simulink model "untitled5"  (R2019b)
settings: Solver=VariableStepAuto  StartTime=0.0  StopTime=5  RelTol=1e-3
model workspace (MAT data in the model file):
  A = Simulink.Signal
  A.DataType = 'double'
  A.Min = 0
  A.Dimensions = 1
  A.DimensionsMode = 'auto'
  A.Complexity = 'auto'
  A.SampleTime = -1
  A.SamplingMode = 'auto'
  A.InitialValue = '0'
values from neighbouring files (symbols this model uses):
  Brad = 0.17    [lab6.m]    (also in multiple_V.m)
  J = 0.0023    [lab6.m]    (also in multiple_V.m)
  Ke = Km    (= 0.29)    [lab6.m]    (also in multiple_V.m)
  Km = 0.29    [lab6.m]    (also in multiple_V.m)
  Kr = 100    [lab6.m]    (also in multiple_V.m)
  Ks = 150    [lab6.m]    (also in multiple_V.m)
  L = 0.0047    [lab6.m]    (also in multiple_V.m)
  R = 4.7    [lab6.m]    (also in multiple_V.m)
  Rad = 0.0275    [lab6.m]    (also in multiple_V.m)
  Um = 3.5    [lab6.m]    (also in multiple_V.m)
settings Model: Creator=Ivan  LastModifiedBy=Ivan
settings SolverCC: AlgebraicLoopSolver=LineSearch

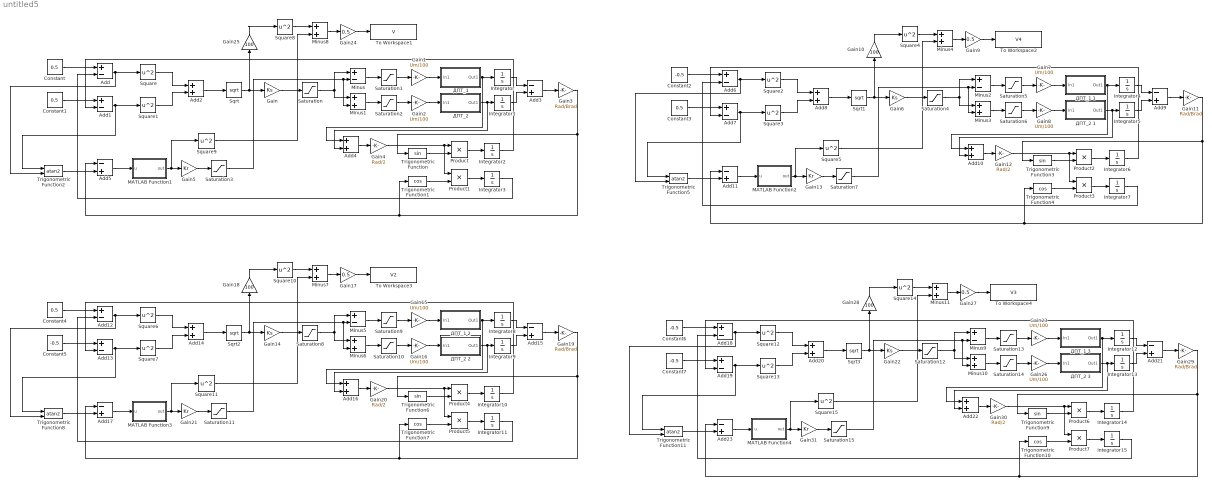
== system untitled5 ==
  Add{,1,6..7,12..13,18..19} (8 alike) : Sum  Inputs=+-
  Add{2,4,8,10,14,16,20,22} (8 alike) : Sum
  Add{3,5,9,11,15,17,21,23} (8 alike) : Sum  Inputs=-+
  Constant{,1,3..4} (4 alike) : Constant  Value=0.5
  Constant{2,5..7} (4 alike) : Constant  Value=-0.5
  Gain{,6,14,22} (4 alike) : Gain  Gain=Ks
  Gain{1..2,7..8,15..16,23,26} (8 alike) : Gain  Gain=Um/100
  Gain{10,18,25,28} (4 alike) : Gain  Gain=100
  Gain{3,11,19,29} (4 alike) : Gain  Gain=Rad/Brad
  Gain{4,12,20,30} (4 alike) : Gain  Gain=Rad/2
  Gain{5,13,21,31} (4 alike) : Gain  Gain=Kr
  Gain{9,17,24,27} (4 alike) : Gain  Gain=0.5
  Integrator{,1..15} (16 alike) : Integrator
  MATLAB Function1 : MATLAB Function  TreatAsAtomicUnit=on  VariantControl=Variant1
  MATLAB Function2 : MATLAB Function  TreatAsAtomicUnit=on  VariantControl=Variant1
  MATLAB Function3 : MATLAB Function  TreatAsAtomicUnit=on  VariantControl=Variant1
  MATLAB Function4 : MATLAB Function  TreatAsAtomicUnit=on  VariantControl=Variant1
  Minus{,2,5,9} (4 alike) : Sum  Inputs=+-
  Minus{1,3..4,6..8,10..11} (8 alike) : Sum
  Product{,1..7} (8 alike) : Product
  Saturation{,4,8,12} (4 alike) : Saturate  UpperLimit=80  LowerLimit=-80
  Saturation{1..2,5..6,9..10,13..14} (8 alike) : Saturate  UpperLimit=100  LowerLimit=-100
  Saturation{3,7,11,15} (4 alike) : Saturate  UpperLimit=20  LowerLimit=-20
  Sqrt{,1..3} (4 alike) : Sqrt  SaturateOnIntegerOverflow=on
  Square{,1..15} (16 alike) : Math  Operator=square  SignedPower=off  SaturateOnIntegerOverflow=on
  To Workspace1 : ToWorkspace  VariableName=V  SaveFormat=Timeseries  SampleTime=-1
  To Workspace2 : ToWorkspace  VariableName=V4  SaveFormat=Timeseries  SampleTime=-1
  To Workspace3 : ToWorkspace  VariableName=V2  SaveFormat=Timeseries  SampleTime=-1
  To Workspace4 : ToWorkspace  VariableName=V3  SaveFormat=Timeseries  SampleTime=-1
  Trigonometric Function{,3,6,9} (4 alike) : Trigonometry
  Trigonometric Function{1,4,7,10} (4 alike) : Trigonometry  Operator=cos
  Trigonometric Function{2,5,8,11} (4 alike) : Trigonometry  Operator=atan2
  "ДПТ_1 " : Subsystem
  ДПТ_1 1 : Subsystem
  ДПТ_1 2 : Subsystem
  ДПТ_1 3 : Subsystem
  "ДПТ_2 " : Subsystem
  ДПТ_2 1 : Subsystem
  ДПТ_2 2 : Subsystem
  ДПТ_2 3 : Subsystem
  wires:
  Add/1 -> Trigonometric Function2/2, Square/1
  Add1/1 -> Trigonometric Function2/1, Square1/1
  Square/1 -> Add2/1
  Square1/1 -> Add2/2
  Add2/1 -> Sqrt/1
  Sqrt/1 -> Gain25/1, Gain/1
  Gain/1 -> Saturation/1
  Saturation/1 -> Minus/1, Minus1/1
  Minus/1 -> Saturation1/1
  Minus1/1 -> Saturation2/1
  Saturation1/1 -> Gain1/1
  Saturation2/1 -> Gain2/1
  Gain1/1 -> "ДПТ_1 "/1(In1)
  Gain2/1 -> "ДПТ_2 "/1(In1)
  "ДПТ_1 "/1(Out1) -> Add4/1, Integrator/1
  "ДПТ_2 "/1(Out1) -> Add4/2, Integrator1/1
  Integrator/1 -> Add3/1
  Integrator1/1 -> Add3/2
  Add3/1 -> Gain3/1
  Add4/1 -> Gain4/1
  Gain4/1 -> Product1/1, Product/1
  Gain3/1 -> Trigonometric Function/1, Trigonometric Function1/1, Add5/1
  Trigonometric Function/1 -> Product/2
  Trigonometric Function1/1 -> Product1/2
  Product/1 -> Integrator2/1
  Product1/1 -> Integrator3/1
  Trigonometric Function2/1 -> Add5/2
  Gain5/1 -> Saturation3/1
  Saturation3/1 -> Minus1/2, Minus/2
  Integrator2/1 -> Add1/2
  Integrator3/1 -> Add/2
  Add5/1 -> MATLAB Function1/1(u)
  MATLAB Function1/1(out) -> Square9/1, Gain5/1
  Constant/1 -> Add/1
  Constant1/1 -> Add1/1
  Minus8/1 -> Gain24/1
  Gain24/1 -> To Workspace1/1
  Square8/1 -> Minus8/1
  Gain25/1 -> Square8/1
  Square9/1 -> Minus8/2
  Constant3/1 -> Add7/1
  Gain9/1 -> To Workspace2/1
  Trigonometric Function3/1 -> Product2/2
  Add9/1 -> Gain11/1
  Add11/1 -> MATLAB Function2/1(u)
  MATLAB Function2/1(out) -> Square5/1, Gain13/1
  Constant2/1 -> Add6/1
  Trigonometric Function4/1 -> Product3/2
  Gain6/1 -> Saturation4/1
  Integrator4/1 -> Add9/1
  Trigonometric Function5/1 -> Add11/2
  Gain13/1 -> Saturation7/1
  Integrator7/1 -> Add6/2
  Gain10/1 -> Square4/1
  Saturation6/1 -> Gain8/1
  Integrator5/1 -> Add9/2
  Add7/1 -> Trigonometric Function5/1, Square3/1
  Gain12/1 -> Product3/1, Product2/1
  Product2/1 -> Integrator6/1
  ДПТ_1 1/1(Out1) -> Add10/1, Integrator4/1
  Gain8/1 -> ДПТ_2 1/1(In1)
  Add10/1 -> Gain12/1
  Square4/1 -> Minus4/1
  ДПТ_2 1/1(Out1) -> Add10/2, Integrator5/1
  Minus2/1 -> Saturation5/1
  Add8/1 -> Sqrt1/1
  Sqrt1/1 -> Gain10/1, Gain6/1
  Minus3/1 -> Saturation6/1
  Gain11/1 -> Trigonometric Function3/1, Trigonometric Function4/1, Add11/1
  Add6/1 -> Trigonometric Function5/2, Square2/1
  Square2/1 -> Add8/1
  Saturation4/1 -> Minus2/1, Minus3/1
  Saturation5/1 -> Gain7/1
  Gain7/1 -> ДПТ_1 1/1(In1)
  Minus4/1 -> Gain9/1
  Saturation7/1 -> Minus3/2, Minus2/2
  Square5/1 -> Minus4/2
  Square3/1 -> Add8/2
  Integrator6/1 -> Add7/2
  Product3/1 -> Integrator7/1
  Constant5/1 -> Add13/1
  Gain17/1 -> To Workspace3/1
  Trigonometric Function6/1 -> Product4/2
  Add15/1 -> Gain19/1
  Add17/1 -> MATLAB Function3/1(u)
  MATLAB Function3/1(out) -> Square11/1, Gain21/1
  Constant4/1 -> Add12/1
  Trigonometric Function7/1 -> Product5/2
  Gain14/1 -> Saturation8/1
  Integrator8/1 -> Add15/1
  Trigonometric Function8/1 -> Add17/2
  Gain21/1 -> Saturation11/1
  Integrator11/1 -> Add12/2
  Gain18/1 -> Square10/1
  Saturation10/1 -> Gain16/1
  Integrator9/1 -> Add15/2
  Add13/1 -> Trigonometric Function8/1, Square7/1
  Gain20/1 -> Product5/1, Product4/1
  Product4/1 -> Integrator10/1
  ДПТ_1 2/1(Out1) -> Add16/1, Integrator8/1
  Gain16/1 -> ДПТ_2 2/1(In1)
  Add16/1 -> Gain20/1
  Square10/1 -> Minus7/1
  ДПТ_2 2/1(Out1) -> Add16/2, Integrator9/1
  Minus5/1 -> Saturation9/1
  Add14/1 -> Sqrt2/1
  Sqrt2/1 -> Gain18/1, Gain14/1
  Minus6/1 -> Saturation10/1
  Gain19/1 -> Trigonometric Function6/1, Trigonometric Function7/1, Add17/1
  Add12/1 -> Trigonometric Function8/2, Square6/1
  Square6/1 -> Add14/1
  Saturation8/1 -> Minus5/1, Minus6/1
  Saturation9/1 -> Gain15/1
  Gain15/1 -> ДПТ_1 2/1(In1)
  Minus7/1 -> Gain17/1
  Saturation11/1 -> Minus6/2, Minus5/2
  Square11/1 -> Minus7/2
  Square7/1 -> Add14/2
  Integrator10/1 -> Add13/2
  Product5/1 -> Integrator11/1
  Constant7/1 -> Add19/1
  Gain27/1 -> To Workspace4/1
  Trigonometric Function9/1 -> Product6/2
  Add21/1 -> Gain29/1
  Add23/1 -> MATLAB Function4/1(u)
  MATLAB Function4/1(out) -> Square15/1, Gain31/1
  Constant6/1 -> Add18/1
  Trigonometric Function10/1 -> Product7/2
  Gain22/1 -> Saturation12/1
  Integrator12/1 -> Add21/1
  Trigonometric Function11/1 -> Add23/2
  Gain31/1 -> Saturation15/1
  Integrator15/1 -> Add18/2
  Gain28/1 -> Square14/1
  Saturation14/1 -> Gain26/1
  Integrator13/1 -> Add21/2
  Add19/1 -> Trigonometric Function11/1, Square13/1
  Gain30/1 -> Product7/1, Product6/1
  Product6/1 -> Integrator14/1
  ДПТ_1 3/1(Out1) -> Add22/1, Integrator12/1
  Gain26/1 -> ДПТ_2 3/1(In1)
  Add22/1 -> Gain30/1
  Square14/1 -> Minus11/1
  ДПТ_2 3/1(Out1) -> Add22/2, Integrator13/1
  Minus9/1 -> Saturation13/1
  Add20/1 -> Sqrt3/1
  Sqrt3/1 -> Gain28/1, Gain22/1
  Minus10/1 -> Saturation14/1
  Gain29/1 -> Trigonometric Function9/1, Trigonometric Function10/1, Add23/1
  Add18/1 -> Trigonometric Function11/2, Square12/1
  Square12/1 -> Add20/1
  Saturation12/1 -> Minus9/1, Minus10/1
  Saturation13/1 -> Gain23/1
  Gain23/1 -> ДПТ_1 3/1(In1)
  Minus11/1 -> Gain27/1
  Saturation15/1 -> Minus10/2, Minus9/2
  Square15/1 -> Minus11/2
  Square13/1 -> Add20/2
  Integrator14/1 -> Add19/2
  Product7/1 -> Integrator15/1

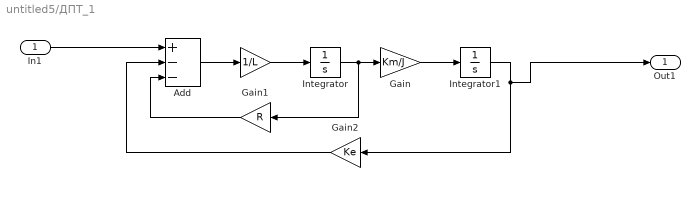
== system untitled5/ДПТ_1  ==
  In1 : Inport
  " " : Gain  Gain=1/L
  Add : Sum  Inputs=+--
  Gain : Gain  Gain=Km/J
  Gain1 : Gain  Gain=R
  Gain2 : Gain  Gain=Ke
  Integrator : Integrator
  Integrator1 : Integrator
  Out1 : Outport
  wires:
  In1/1 -> Add/1
  Add/1 -> " "/1
  " "/1 -> Integrator/1
  Integrator/1 -> Gain1/1, Gain/1
  Gain/1 -> Integrator1/1
  Integrator1/1 -> Out1/1, Gain2/1
  Gain1/1 -> Add/3
  Gain2/1 -> Add/2

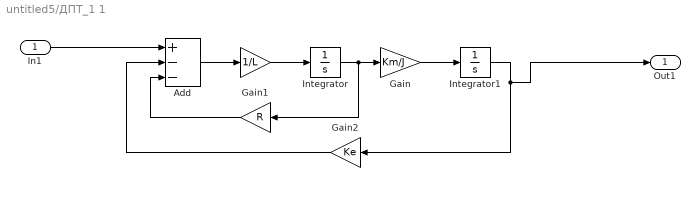
== system untitled5/ДПТ_1 1 ==
  In1 : Inport
  " " : Gain  Gain=1/L
  Add : Sum  Inputs=+--
  Gain : Gain  Gain=Km/J
  Gain1 : Gain  Gain=R
  Gain2 : Gain  Gain=Ke
  Integrator : Integrator
  Integrator1 : Integrator
  Out1 : Outport
  wires:
  In1/1 -> Add/1
  Add/1 -> " "/1
  " "/1 -> Integrator/1
  Integrator/1 -> Gain1/1, Gain/1
  Gain/1 -> Integrator1/1
  Integrator1/1 -> Out1/1, Gain2/1
  Gain1/1 -> Add/3
  Gain2/1 -> Add/2

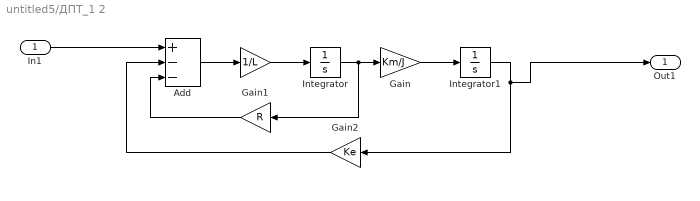
== system untitled5/ДПТ_1 2 ==
  In1 : Inport
  " " : Gain  Gain=1/L
  Add : Sum  Inputs=+--
  Gain : Gain  Gain=Km/J
  Gain1 : Gain  Gain=R
  Gain2 : Gain  Gain=Ke
  Integrator : Integrator
  Integrator1 : Integrator
  Out1 : Outport
  wires:
  In1/1 -> Add/1
  Add/1 -> " "/1
  " "/1 -> Integrator/1
  Integrator/1 -> Gain1/1, Gain/1
  Gain/1 -> Integrator1/1
  Integrator1/1 -> Out1/1, Gain2/1
  Gain1/1 -> Add/3
  Gain2/1 -> Add/2

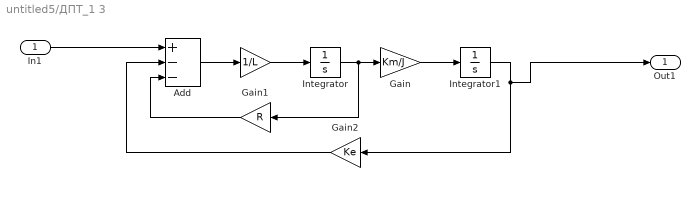
== system untitled5/ДПТ_1 3 ==
  In1 : Inport
  " " : Gain  Gain=1/L
  Add : Sum  Inputs=+--
  Gain : Gain  Gain=Km/J
  Gain1 : Gain  Gain=R
  Gain2 : Gain  Gain=Ke
  Integrator : Integrator
  Integrator1 : Integrator
  Out1 : Outport
  wires:
  In1/1 -> Add/1
  Add/1 -> " "/1
  " "/1 -> Integrator/1
  Integrator/1 -> Gain1/1, Gain/1
  Gain/1 -> Integrator1/1
  Integrator1/1 -> Out1/1, Gain2/1
  Gain1/1 -> Add/3
  Gain2/1 -> Add/2

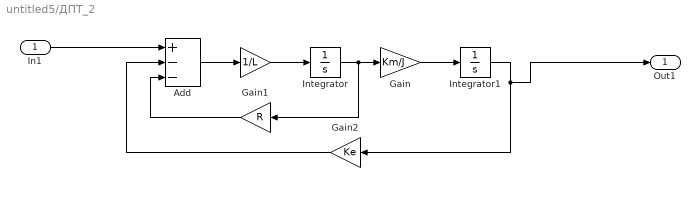
== system untitled5/ДПТ_2  ==
  In1 : Inport
  " " : Gain  Gain=1/L
  Add : Sum  Inputs=+--
  Gain : Gain  Gain=Km/J
  Gain1 : Gain  Gain=R
  Gain2 : Gain  Gain=Ke
  Integrator : Integrator
  Integrator1 : Integrator
  Out1 : Outport
  wires:
  In1/1 -> Add/1
  Add/1 -> " "/1
  " "/1 -> Integrator/1
  Integrator/1 -> Gain1/1, Gain/1
  Gain/1 -> Integrator1/1
  Integrator1/1 -> Out1/1, Gain2/1
  Gain1/1 -> Add/3
  Gain2/1 -> Add/2

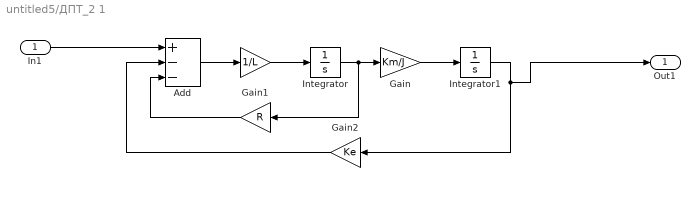
== system untitled5/ДПТ_2 1 ==
  In1 : Inport
  " " : Gain  Gain=1/L
  Add : Sum  Inputs=+--
  Gain : Gain  Gain=Km/J
  Gain1 : Gain  Gain=R
  Gain2 : Gain  Gain=Ke
  Integrator : Integrator
  Integrator1 : Integrator
  Out1 : Outport
  wires:
  In1/1 -> Add/1
  Add/1 -> " "/1
  " "/1 -> Integrator/1
  Integrator/1 -> Gain1/1, Gain/1
  Gain/1 -> Integrator1/1
  Integrator1/1 -> Out1/1, Gain2/1
  Gain1/1 -> Add/3
  Gain2/1 -> Add/2

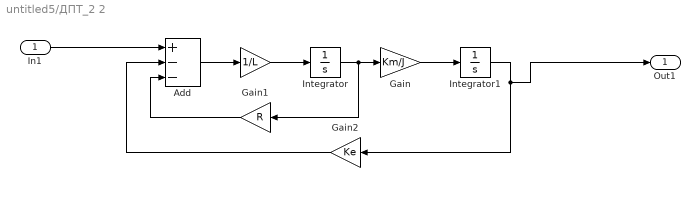
== system untitled5/ДПТ_2 2 ==
  In1 : Inport
  " " : Gain  Gain=1/L
  Add : Sum  Inputs=+--
  Gain : Gain  Gain=Km/J
  Gain1 : Gain  Gain=R
  Gain2 : Gain  Gain=Ke
  Integrator : Integrator
  Integrator1 : Integrator
  Out1 : Outport
  wires:
  In1/1 -> Add/1
  Add/1 -> " "/1
  " "/1 -> Integrator/1
  Integrator/1 -> Gain1/1, Gain/1
  Gain/1 -> Integrator1/1
  Integrator1/1 -> Out1/1, Gain2/1
  Gain1/1 -> Add/3
  Gain2/1 -> Add/2

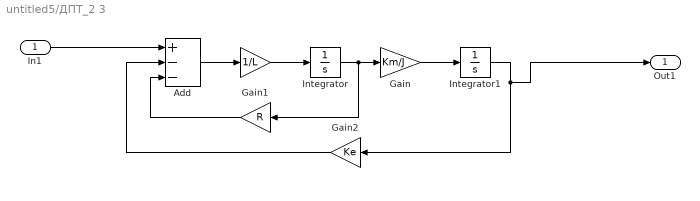
== system untitled5/ДПТ_2 3 ==
  In1 : Inport
  " " : Gain  Gain=1/L
  Add : Sum  Inputs=+--
  Gain : Gain  Gain=Km/J
  Gain1 : Gain  Gain=R
  Gain2 : Gain  Gain=Ke
  Integrator : Integrator
  Integrator1 : Integrator
  Out1 : Outport
  wires:
  In1/1 -> Add/1
  Add/1 -> " "/1
  " "/1 -> Integrator/1
  Integrator/1 -> Gain1/1, Gain/1
  Gain/1 -> Integrator1/1
  Integrator1/1 -> Out1/1, Gain2/1
  Gain1/1 -> Add/3
  Gain2/1 -> Add/2

== matlab function untitled5/MATLAB Function2 ==
  data: u input; out output
function out = fcn(u)
%%codegen
    if (abs(u)>3.14)
        y=u-sign(u)*2*3.14;
    else
        y=u;
    end
out = y;

== matlab function untitled5/MATLAB Function1 ==
  data: u input; out output
function out = fcn(u)
%%codegen
    if (abs(u)>3.14)
        y=u-sign(u)*2*3.14;
    else
        y=u;
    end
out = y;

== matlab function untitled5/MATLAB Function3 ==
  data: u input; out output
function out = fcn(u)
%%codegen
    if (abs(u)>3.14)
        y=u-sign(u)*2*3.14;
    else
        y=u;
    end
out = y;

== matlab function untitled5/MATLAB Function4 ==
  data: u input; out output
function out = fcn(u)
%%codegen
    if (abs(u)>3.14)
        y=u-sign(u)*2*3.14;
    else
        y=u;
    end
out = y;
